simulink model "Main"  (R2024a)
settings: Solver=VariableStepAuto  StartTime=0.0  StopTime=stop_time  RelTol=1e-3
values from neighbouring files (symbols this model uses):
  A_ca = sqrt(2)    [load_params.m]
  c = 299792458    [load_params.m]
  ca_code = generateCAcodes(PRN)    [load_params.m]
  code_repeat = 0.001    [load_params.m]
  data_repeat = 30    [load_params.m]
  df_Dop = 1000    [load_params.m]
  dt_iono = 15E-9    (= 1.5e-08)    [load_params.m]
  dt_rec = 0    [load_params.m]
  dt_sv = 0    [load_params.m]
  dt_tropo = 5E-9    (= 5e-09)    [load_params.m]
  Early_Late = (correlator_spacing * Tc) / 2    (= 4.88758553275e-07)    [load_params.m]
  fB = 1.5E6    (= 1500000)    [load_params.m]
  fb = fB    (= 1500000)    [load_params.m]
  fc = 1.023E6    (= 1023000)    [load_params.m]
  fdata = 50    [load_params.m]
  ferr = f_error    (= 0)    [load_params.m]
  fL1 = 1575.42E6    (= 1575420000)    [load_params.m]
  nav_data = ones(1, 30*50)    [load_params.m]
  perr_rad = phase_error_rad    [load_params.m]
  r_true_t0 = 20E6    (= 20000000)    [load_params.m]
  t_code_bias = code_bias * Tc    (= 0)    [load_params.m]
  Tc = 1 / fc    (= 9.77517106549e-07)    [load_params.m]
  Ts = 1/fs    (= 2.5e-07)    [load_params.m]
undefined symbols (not defined in the file or in its folder): DiscIntNeverNeededParam
libraries: commfilt2 x6, dspsrcs4 x2
settings Model: Creator=Alireza  LastModifiedBy=Alireza

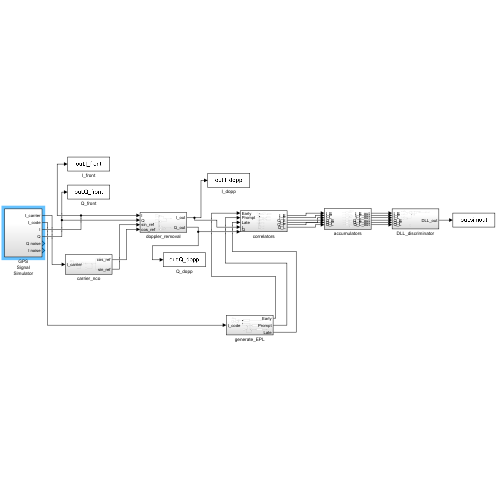
[thumbnail: Simulink's stored preview of the top-level diagram]
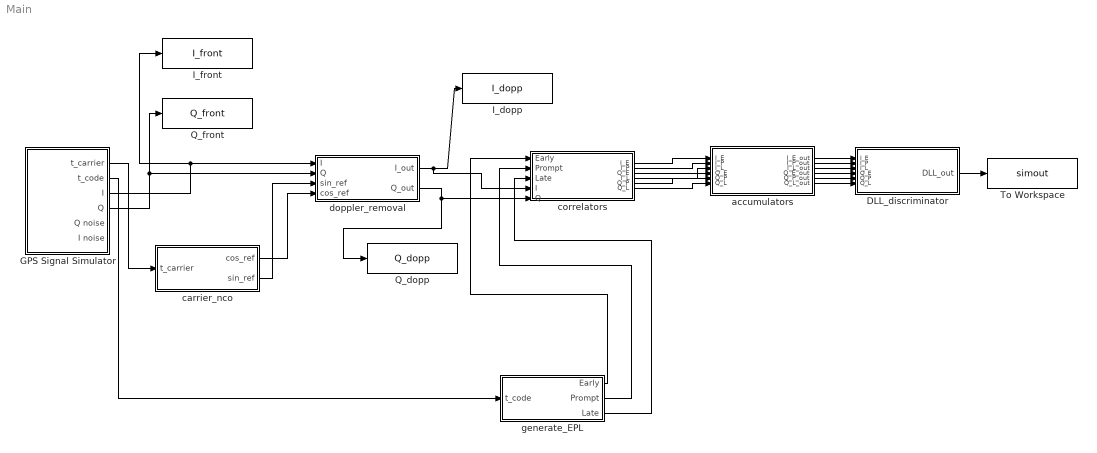
== system Main ==
  DLL_discriminator : Subsystem
  GPS Signal Simulator : Subsystem
  I_dopp : ToWorkspace  VariableName=I_dopp  SampleTime=-1
  I_front : ToWorkspace  VariableName=I_front  SampleTime=-1
  Q_dopp : ToWorkspace  VariableName=Q_dopp  SampleTime=-1
  Q_front : ToWorkspace  VariableName=Q_front  SampleTime=-1
  To Workspace : ToWorkspace  VariableName=simout  SaveFormat=Timeseries  SampleTime=-1
  accumulators : Subsystem
  carrier_nco : Subsystem
  correlators : Subsystem
  doppler_removal : Subsystem
  generate_EPL : Subsystem
  wires:
  carrier_nco/1(cos_ref) -> doppler_removal/4(cos_ref)
  carrier_nco/2(sin_ref) -> doppler_removal/3(sin_ref)
  doppler_removal/1(I_out) -> correlators/4(I), I_dopp/1
  doppler_removal/2(Q_out) -> correlators/5(Q), Q_dopp/1
  GPS Signal Simulator/3(I) -> I_front/1, doppler_removal/1(I)
  GPS Signal Simulator/4(Q) -> Q_front/1, doppler_removal/2(Q)
  GPS Signal Simulator/1(t_carrier) -> carrier_nco/1(t_carrier)
  generate_EPL/1(Early) -> correlators/1(Early)
  generate_EPL/2(Prompt) -> correlators/2(Prompt)
  generate_EPL/3(Late) -> correlators/3(Late)
  correlators/1(I_E) -> accumulators/1(I_E)
  correlators/2(I_P) -> accumulators/2(I_P)
  correlators/4(I_L) -> accumulators/3(I_L)
  correlators/3(Q_E) -> accumulators/4(Q_E)
  correlators/5(Q_P) -> accumulators/5(Q_P)
  correlators/6(Q_L) -> accumulators/6(Q_L)
  accumulators/1(I_E_out) -> DLL_discriminator/1(I_E)
  accumulators/2(I_P_out) -> DLL_discriminator/2(I_P)
  accumulators/3(I_L_out) -> DLL_discriminator/3(I_L)
  accumulators/4(Q_E_out) -> DLL_discriminator/4(Q_E)
  accumulators/5(Q_P_out) -> DLL_discriminator/5(Q_P)
  accumulators/6(Q_L_out) -> DLL_discriminator/6(Q_L)
  DLL_discriminator/1(DLL_out) -> To Workspace/1
  GPS Signal Simulator/2(t_code) -> generate_EPL/1(t_code)

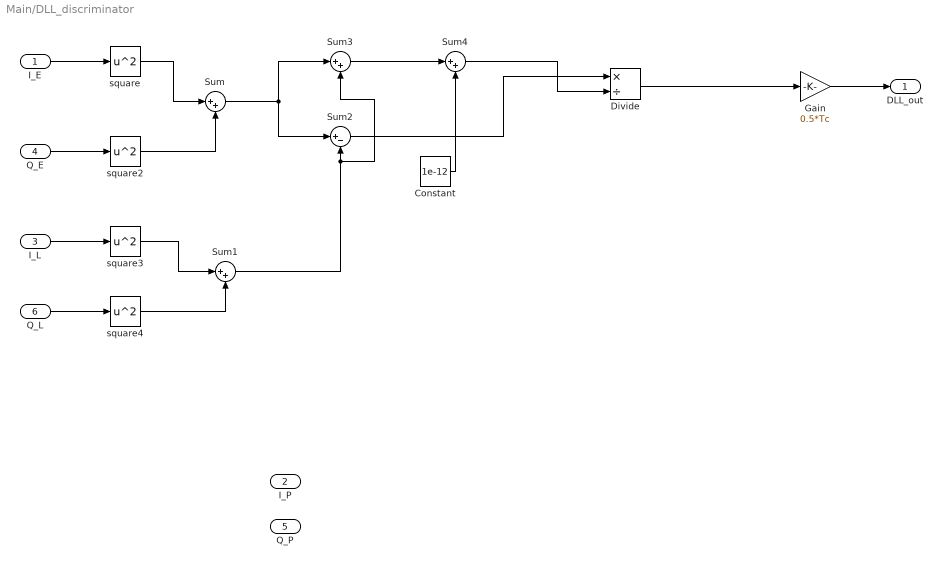
== system Main/DLL_discriminator ==
  I_E : Inport
  I_P : Inport  Port=2
  I_L : Inport  Port=3
  Q_E : Inport  Port=4
  Q_P : Inport  Port=5
  Q_L : Inport  Port=6
  Constant : Constant  Value=1e-12
  Divide : Product  Inputs=*/
  Gain : Gain  Gain=0.5*Tc
  Sum{,1,3..4} (4 alike) : Sum  Inputs=|++
  Sum2 : Sum  Inputs=|+-
  square{,2..4} (4 alike) : Math  Operator=square
  DLL_out : Outport
  wires:
  I_E/1 -> square/1
  Q_E/1 -> square2/1
  square/1 -> Sum/1
  square2/1 -> Sum/2
  Q_L/1 -> square4/1
  I_L/1 -> square3/1
  square3/1 -> Sum1/1
  square4/1 -> Sum1/2
  Sum1/1 -> Sum3/2, Sum2/2
  Sum/1 -> Sum3/1, Sum2/1
  Gain/1 -> DLL_out/1
  Divide/1 -> Gain/1
  Sum2/1 -> Divide/1
  Sum3/1 -> Sum4/1
  Constant/1 -> Sum4/2
  Sum4/1 -> Divide/2

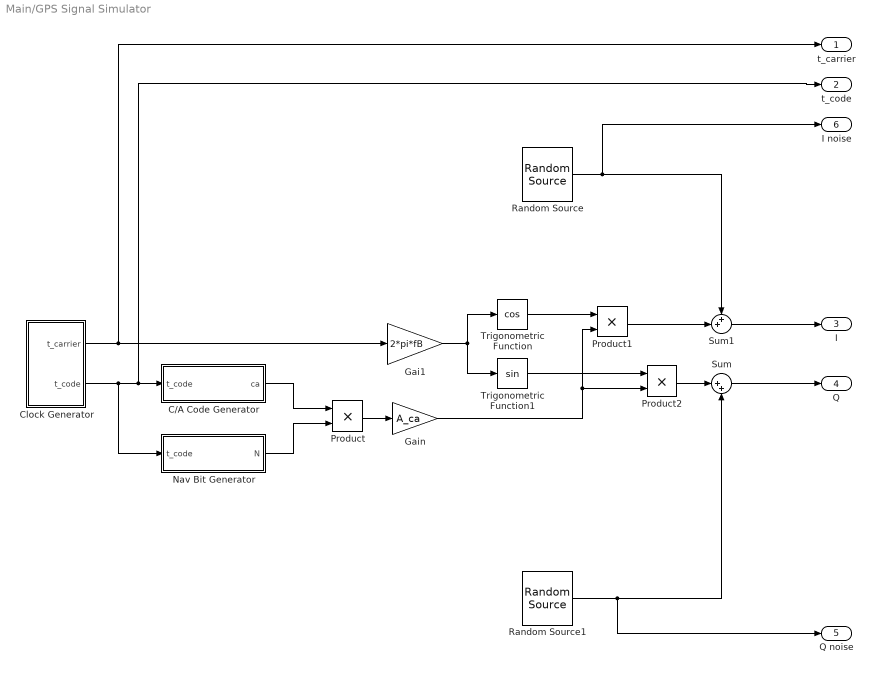
== system Main/GPS Signal Simulator ==
  C/A Code Generator : Subsystem
  Clock Generator : Subsystem
  Gai1 : Gain  Gain=2*pi*fB
  Gain : Gain  Gain=A_ca
  Nav Bit Generator : Subsystem
  Product : Product  RndMeth=Zero
  Product1 : Product  RndMeth=Zero
  Product2 : Product  RndMeth=Zero
  Random Source : dspsrcs4/Random Source  SrcType=Gaussian  MinVal=0  MaxVal=1  MeanVal=0  VarVal=Pn  RepMode=Specify seed  rawSeed=1  IsInherit=off  SampTime=Ts  SampFrame=1  OutComplex=Real  DataType=double  SimulateUsing=Interpreted execution
  Random Source1 : dspsrcs4/Random Source  SrcType=Gaussian  MinVal=0  MaxVal=1  MeanVal=0  VarVal=Pn  RepMode=Specify seed  rawSeed=2  IsInherit=off  SampTime=Ts  SampFrame=1  OutComplex=Real  DataType=double  SimulateUsing=Interpreted execution
  Sum : Sum  Inputs=|++
  Sum1 : Sum  Inputs=++|
  Trigonometric Function : Trigonometry  Operator=cos
  Trigonometric Function1 : Trigonometry
  t_carrier : Outport
  t_code : Outport  Port=2
  I : Outport  Port=3
  Q : Outport  Port=4
  Q noise : Outport  Port=5
  I noise : Outport  Port=6
  wires:
  Clock Generator/2(t_code) -> Nav Bit Generator/1(t_code), C/A Code Generator/1(t_code), t_code/1
  C/A Code Generator/1(ca) -> Product/1
  Nav Bit Generator/1(N) -> Product/2
  Product/1 -> Gain/1
  Clock Generator/1(t_carrier) -> Gai1/1, t_carrier/1
  Gai1/1 -> Trigonometric Function1/1, Trigonometric Function/1
  Gain/1 -> Product1/2, Product2/2
  Trigonometric Function/1 -> Product1/1
  Trigonometric Function1/1 -> Product2/1
  Random Source1/1 -> Sum/2, Q noise/1
  Random Source/1 -> Sum1/1, I noise/1
  Sum/1 -> Q/1
  Sum1/1 -> I/1
  Product1/1 -> Sum1/2
  Product2/1 -> Sum/1

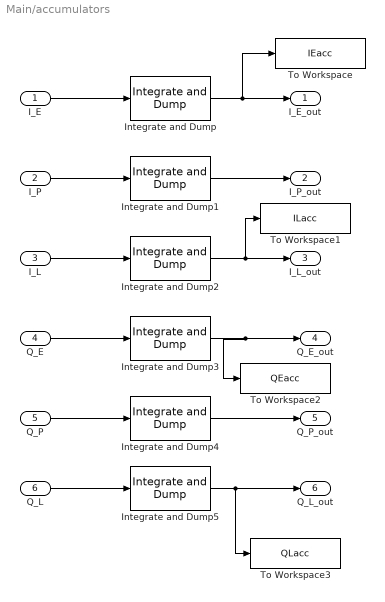
== system Main/accumulators ==
  I_E : Inport
  I_P : Inport  Port=2
  I_L : Inport  Port=3
  Q_E : Inport  Port=4
  Q_P : Inport  Port=5
  Q_L : Inport  Port=6
  Integrate and Dump{,1..5} (6 alike) : commfilt2/Integrate and Dump  obssamples=ME  offsetsamples=0  nodump=off  roundingMode=Floor  overflowMode=off  outputDataTypeStr=Inherit: Same as accumulator  outputLastDataTypeStr=Inherit: Same as accumulator
  To Workspace : ToWorkspace  VariableName=IEacc  SaveFormat=Timeseries  SampleTime=-1
  To Workspace1 : ToWorkspace  VariableName=ILacc  SaveFormat=Timeseries  SampleTime=-1
  To Workspace2 : ToWorkspace  VariableName=QEacc  SaveFormat=Timeseries  SampleTime=-1
  To Workspace3 : ToWorkspace  VariableName=QLacc  SaveFormat=Timeseries  SampleTime=-1
  I_E_out : Outport
  I_P_out : Outport  Port=2
  I_L_out : Outport  Port=3
  Q_E_out : Outport  Port=4
  Q_P_out : Outport  Port=5
  Q_L_out : Outport  Port=6
  wires:
  I_E/1 -> Integrate and Dump/1
  Integrate and Dump/1 -> To Workspace/1, I_E_out/1
  I_P/1 -> Integrate and Dump1/1
  Integrate and Dump1/1 -> I_P_out/1
  I_L/1 -> Integrate and Dump2/1
  Integrate and Dump2/1 -> To Workspace1/1, I_L_out/1
  Q_E/1 -> Integrate and Dump3/1
  Integrate and Dump3/1 -> To Workspace2/1, Q_E_out/1
  Q_P/1 -> Integrate and Dump4/1
  Integrate and Dump4/1 -> Q_P_out/1
  Q_L/1 -> Integrate and Dump5/1
  Integrate and Dump5/1 -> To Workspace3/1, Q_L_out/1

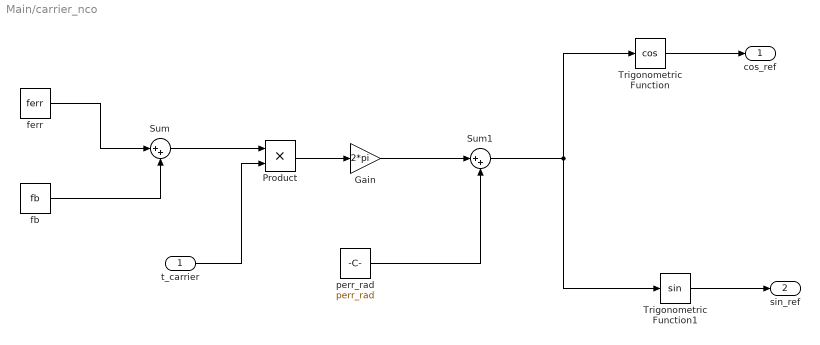
== system Main/carrier_nco ==
  t_carrier : Inport
  Gain : Gain  Gain=2*pi
  Product : Product
  Sum : Sum  Inputs=|++
  Sum1 : Sum  Inputs=|++
  Trigonometric Function : Trigonometry  Operator=cos
  Trigonometric Function1 : Trigonometry
  fb : Constant  Value=fb
  ferr : Constant  Value=ferr
  perr_rad : Constant  Value=perr_rad
  cos_ref : Outport
  sin_ref : Outport  Port=2
  wires:
  Trigonometric Function1/1 -> sin_ref/1
  t_carrier/1 -> Product/2
  Sum1/1 -> Trigonometric Function1/1, Trigonometric Function/1
  Trigonometric Function/1 -> cos_ref/1
  perr_rad/1 -> Sum1/2
  Gain/1 -> Sum1/1
  fb/1 -> Sum/2
  Product/1 -> Gain/1
  ferr/1 -> Sum/1
  Sum/1 -> Product/1

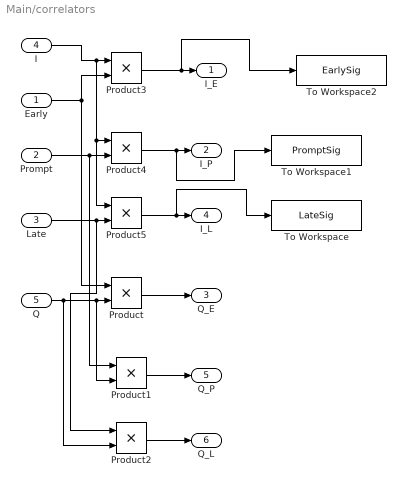
== system Main/correlators ==
  Early : Inport
  Prompt : Inport  Port=2
  Late : Inport  Port=3
  I : Inport  Port=4
  Q : Inport  Port=5
  Product{,1..5} (6 alike) : Product
  To Workspace : ToWorkspace  VariableName=LateSig  SaveFormat=Timeseries  SampleTime=-1
  To Workspace1 : ToWorkspace  VariableName=PromptSig  SaveFormat=Timeseries  SampleTime=-1
  To Workspace2 : ToWorkspace  VariableName=EarlySig  SaveFormat=Timeseries  SampleTime=-1
  I_E : Outport
  I_P : Outport  Port=2
  Q_E : Outport  Port=3
  I_L : Outport  Port=4
  Q_P : Outport  Port=5
  Q_L : Outport  Port=6
  wires:
  I/1 -> Product4/1, Product5/1, Product3/1
  Early/1 -> Product/1, Product3/2
  Product3/1 -> To Workspace2/1, I_E/1
  Prompt/1 -> Product4/2, Product1/1
  Product4/1 -> To Workspace1/1, I_P/1
  Late/1 -> Product2/1, Product5/2
  Product5/1 -> To Workspace/1, I_L/1
  Q/1 -> Product2/2, Product1/2, Product/2
  Product/1 -> Q_E/1
  Product1/1 -> Q_P/1
  Product2/1 -> Q_L/1

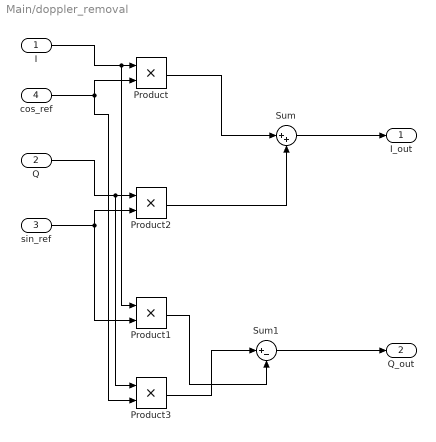
== system Main/doppler_removal ==
  I : Inport
  Q : Inport  Port=2
  sin_ref : Inport  Port=3
  cos_ref : Inport  Port=4
  Product{,1..3} (4 alike) : Product
  Sum : Sum  Inputs=|++
  Sum1 : Sum  Inputs=|+-
  I_out : Outport
  Q_out : Outport  Port=2
  wires:
  I/1 -> Product1/1, Product/1
  cos_ref/1 -> Product3/2, Product/2
  Q/1 -> Product2/1, Product3/1
  sin_ref/1 -> Product1/2, Product2/2
  Product/1 -> Sum/1
  Product2/1 -> Sum/2
  Sum/1 -> I_out/1
  Sum1/1 -> Q_out/1
  Product3/1 -> Sum1/1
  Product1/1 -> Sum1/2

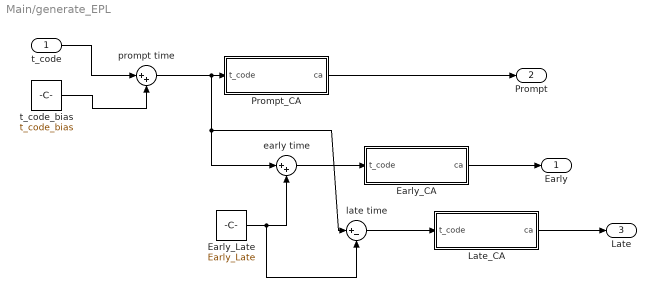
== system Main/generate_EPL ==
  t_code : Inport
  Early_CA : Subsystem
  Early_Late : Constant  Value=Early_Late
  Late_CA : Subsystem
  Prompt_CA : Subsystem
  early time : Sum  Inputs=|++
  late time : Sum  Inputs=|+-
  prompt time : Sum  Inputs=|++
  t_code_bias : Constant  Value=t_code_bias
  Early : Outport
  Prompt : Outport  Port=2
  Late : Outport  Port=3
  wires:
  t_code/1 -> prompt time/1
  t_code_bias/1 -> prompt time/2
  prompt time/1 -> early time/1, late time/1, Prompt_CA/1(t_code)
  Early_Late/1 -> late time/2, early time/2
  early time/1 -> Early_CA/1(t_code)
  late time/1 -> Late_CA/1(t_code)
  Late_CA/1(ca) -> Late/1
  Prompt_CA/1(ca) -> Prompt/1
  Early_CA/1(ca) -> Early/1

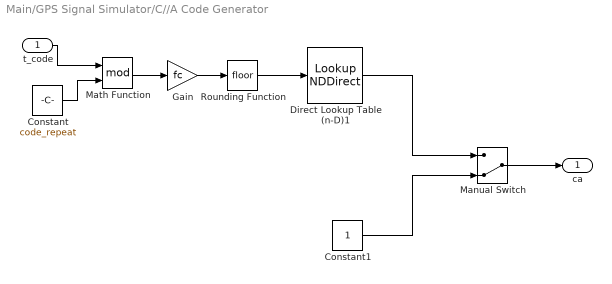
== system Main/GPS Signal Simulator/C//A Code Generator ==
  t_code : Inport
  Constant : Constant  Value=code_repeat
  Constant1 : Constant
  Direct Lookup Table (n-D)1 : LookupNDDirect  NumberOfTableDimensions=1  Table=ca_code
  Gain : Gain  Gain=fc
  Manual Switch : ManualSwitch  CurrentSetting=0
  Math Function : Math  Operator=mod  SignedPower=on
  Rounding Function : Rounding
  ca : Outport
  wires:
  Constant/1 -> Math Function/2
  Math Function/1 -> Gain/1
  Gain/1 -> Rounding Function/1
  Rounding Function/1 -> Direct Lookup Table (n-D)1/1
  t_code/1 -> Math Function/1
  Direct Lookup Table (n-D)1/1 -> Manual Switch/1
  Constant1/1 -> Manual Switch/2
  Manual Switch/1 -> ca/1

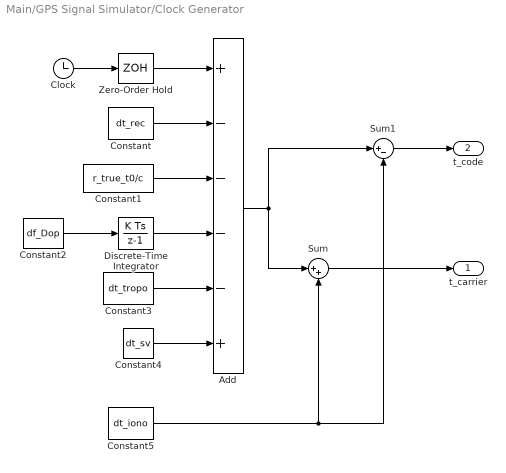
== system Main/GPS Signal Simulator/Clock Generator ==
  Add : Sum  Inputs=+----+
  Clock : Clock
  Constant : Constant  Value=dt_rec
  Constant1 : Constant  Value=r_true_t0/c
  Constant2 : Constant  Value=df_Dop
  Constant3 : Constant  Value=dt_tropo
  Constant4 : Constant  Value=dt_sv
  Constant5 : Constant  Value=dt_iono
  Discrete-Time Integrator : DiscreteIntegrator  gainval=1/fL1  SampleTime=Ts  ICPrevOutput=DiscIntNeverNeededParam  ICPrevScaledInput=DiscIntNeverNeededParam
  Sum : Sum  Inputs=|++
  Sum1 : Sum  Inputs=|+-
  Zero-Order Hold : ZeroOrderHold  SampleTime=Ts
  t_carrier : Outport
  t_code : Outport  Port=2
  wires:
  Clock/1 -> Zero-Order Hold/1
  Constant/1 -> Add/2
  Constant1/1 -> Add/3
  Constant2/1 -> Discrete-Time Integrator/1
  Discrete-Time Integrator/1 -> Add/4
  Constant3/1 -> Add/5
  Zero-Order Hold/1 -> Add/1
  Constant4/1 -> Add/6
  Add/1 -> Sum/1, Sum1/1
  Constant5/1 -> Sum/2, Sum1/2
  Sum1/1 -> t_code/1
  Sum/1 -> t_carrier/1

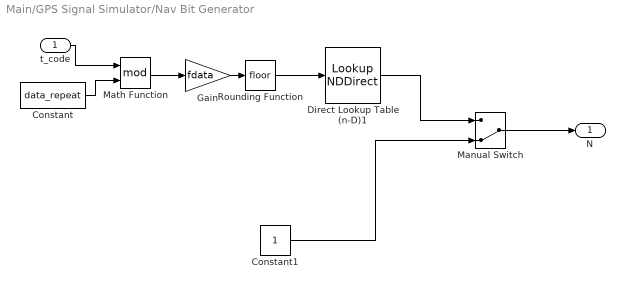
== system Main/GPS Signal Simulator/Nav Bit Generator ==
  t_code : Inport
  Constant : Constant  Value=data_repeat
  Constant1 : Constant
  Direct Lookup Table (n-D)1 : LookupNDDirect  NumberOfTableDimensions=1  Table=nav_data
  Gain : Gain  Gain=fdata
  Manual Switch : ManualSwitch  CurrentSetting=0
  Math Function : Math  Operator=mod  SignedPower=on
  Rounding Function : Rounding
  N : Outport
  wires:
  Constant/1 -> Math Function/2
  Math Function/1 -> Gain/1
  Gain/1 -> Rounding Function/1
  Rounding Function/1 -> Direct Lookup Table (n-D)1/1
  t_code/1 -> Math Function/1
  Direct Lookup Table (n-D)1/1 -> Manual Switch/1
  Constant1/1 -> Manual Switch/2
  Manual Switch/1 -> N/1

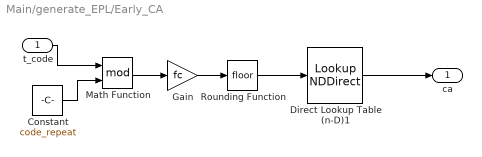
== system Main/generate_EPL/Early_CA ==
  t_code : Inport
  Constant : Constant  Value=code_repeat
  Direct Lookup Table (n-D)1 : LookupNDDirect  NumberOfTableDimensions=1  Table=ca_code
  Gain : Gain  Gain=fc
  Math Function : Math  Operator=mod  SignedPower=on
  Rounding Function : Rounding
  ca : Outport
  wires:
  Constant/1 -> Math Function/2
  Math Function/1 -> Gain/1
  Gain/1 -> Rounding Function/1
  Rounding Function/1 -> Direct Lookup Table (n-D)1/1
  t_code/1 -> Math Function/1
  Direct Lookup Table (n-D)1/1 -> ca/1

== system Main/generate_EPL/Late_CA ==
  t_code : Inport
  Constant : Constant  Value=code_repeat
  Direct Lookup Table (n-D)1 : LookupNDDirect  NumberOfTableDimensions=1  Table=ca_code
  Gain : Gain  Gain=fc
  Math Function : Math  Operator=mod  SignedPower=on
  Rounding Function : Rounding
  ca : Outport
  wires:
  Constant/1 -> Math Function/2
  Math Function/1 -> Gain/1
  Gain/1 -> Rounding Function/1
  Rounding Function/1 -> Direct Lookup Table (n-D)1/1
  t_code/1 -> Math Function/1
  Direct Lookup Table (n-D)1/1 -> ca/1

== system Main/generate_EPL/Prompt_CA ==
  t_code : Inport
  Constant : Constant  Value=code_repeat
  Direct Lookup Table (n-D)1 : LookupNDDirect  NumberOfTableDimensions=1  Table=ca_code
  Gain : Gain  Gain=fc
  Math Function : Math  Operator=mod  SignedPower=on
  Rounding Function : Rounding
  ca : Outport
  wires:
  Constant/1 -> Math Function/2
  Math Function/1 -> Gain/1
  Gain/1 -> Rounding Function/1
  Rounding Function/1 -> Direct Lookup Table (n-D)1/1
  t_code/1 -> Math Function/1
  Direct Lookup Table (n-D)1/1 -> ca/1
